simulink model "Realizacion_Retroalimentacion_Estados"  (R2023b)
settings: Solver=ode4  StartTime=0.0  StopTime=15  FixedStep=0.01  RelTol=1e-3
values from neighbouring files (symbols this model uses):
  Gf = feedback(G1*G2,H)    [Exp1_Realizacion.m]
  K = place(A,B,pcc)    [Exp1_Realizacion.m]
  Ke = Ke'    [Exp1_Realizacion.m]
undefined symbols (not defined in the file or in its folder): A, B, C, D
settings Model: Creator=carlo  LastModifiedBy=carlo

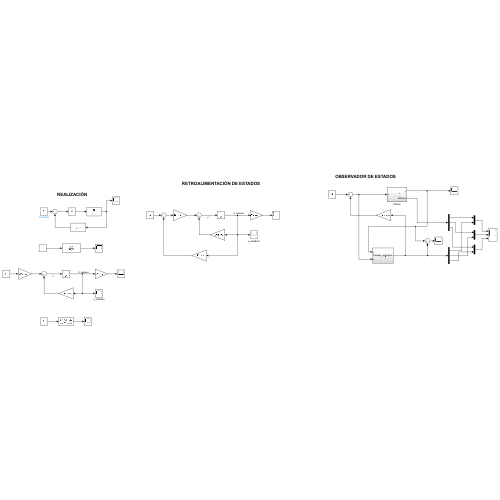
[thumbnail: Simulink's stored preview of the top-level diagram]
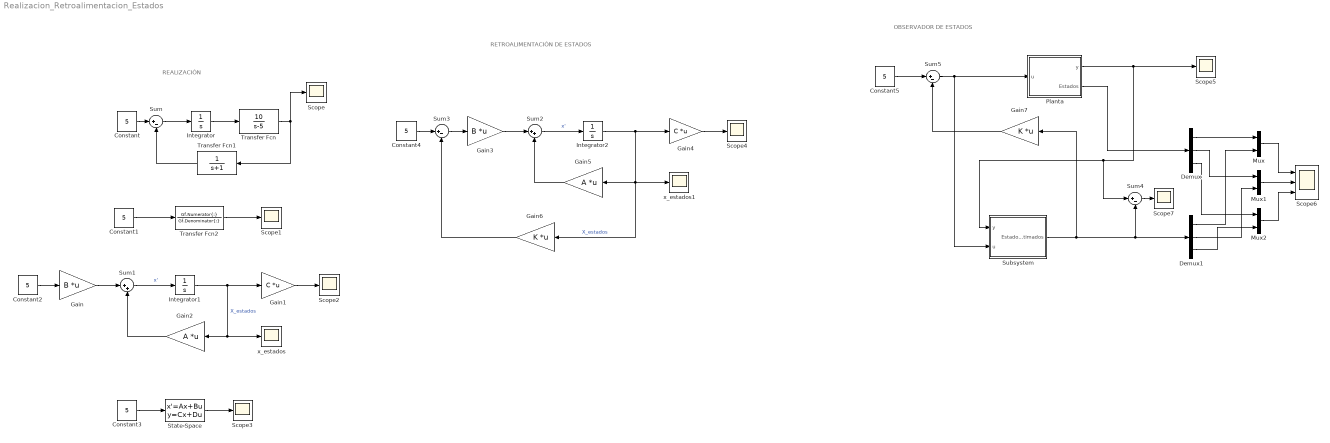
== system Realizacion_Retroalimentacion_Estados ==
  note: REALIZACIÓN
  note: RETROALIMENTACIÓN DE ESTADOS
  note: OBSERVADOR DE ESTADOS
  Constant{,1..5} (6 alike) : Constant  Value=5
  Demux : Demux  Outputs=3
  Demux1 : Demux  Outputs=3
  Gain : Gain  Gain=B  Multiplication=Matrix(K*u) (u vector)
  Gain1 : Gain  Gain=C  Multiplication=Matrix(K*u) (u vector)
  Gain2 : Gain  Gain=A  Multiplication=Matrix(K*u) (u vector)
  Gain3 : Gain  Gain=B  Multiplication=Matrix(K*u) (u vector)
  Gain4 : Gain  Gain=C  Multiplication=Matrix(K*u) (u vector)
  Gain5 : Gain  Gain=A  Multiplication=Matrix(K*u) (u vector)
  Gain6 : Gain  Gain=K  Multiplication=Matrix(K*u) (u vector)
  Gain7 : Gain  Gain=K  Multiplication=Matrix(K*u) (u vector)
  Integrator : Integrator
  Integrator1 : Integrator  InitialCondition=[2 4 7]'
  Integrator2 : Integrator  InitialCondition=[5 -4 7]'
  Mux : Mux  Inputs=2
  Mux1 : Mux  Inputs=2
  Mux2 : Mux  Inputs=2
  Planta : Subsystem
  Scope{,1..5,7} (7 alike) : Scope
  Scope6 : Scope  NumInputPorts=3
  State-Space : StateSpace  A=A  B=B  C=C  D=D  InitialCondition=[3 0 0]'
  Subsystem : Subsystem
  Sum{,3..5} (4 alike) : Sum  Inputs=|+-
  Sum1 : Sum  Inputs=|++
  Sum2 : Sum  Inputs=|++
  Transfer Fcn : TransferFcn  Numerator=[10]  Denominator=[1 -5]
  Transfer Fcn1 : TransferFcn  Denominator=[1 1]
  Transfer Fcn2 : TransferFcn  Numerator=Gf.Numerator{:}  Denominator=Gf.Denominator{:}
  x_estados : Scope
  x_estados1 : Scope
  wires:
  Constant/1 -> Sum/1
  Sum/1 -> Integrator/1
  Integrator/1 -> Transfer Fcn/1
  Transfer Fcn/1 -> Scope/1, Transfer Fcn1/1
  Transfer Fcn1/1 -> Sum/2
  Constant1/1 -> Transfer Fcn2/1
  Transfer Fcn2/1 -> Scope1/1
  Gain2/1 -> Sum1/2
  Integrator1/1 -> x_estados/1, Gain2/1, Gain1/1  "X_estados"
  Gain/1 -> Sum1/1
  Sum1/1 -> Integrator1/1  "x'"
  Constant2/1 -> Gain/1
  Gain1/1 -> Scope2/1
  Constant3/1 -> State-Space/1
  State-Space/1 -> Scope3/1
  Gain4/1 -> Scope4/1
  Sum2/1 -> Integrator2/1  "x'"
  Gain3/1 -> Sum2/1
  Integrator2/1 -> Gain4/1, Gain6/1, x_estados1/1, Gain5/1  "X_estados"
  Gain5/1 -> Sum2/2
  Constant4/1 -> Sum3/1
  Sum3/1 -> Gain3/1
  Gain6/1 -> Sum3/2
  Constant5/1 -> Sum5/1
  Sum5/1 -> Subsystem/2(u), Planta/1(u)
  Planta/1(y) -> Sum4/1, Subsystem/1(y), Scope5/1
  Subsystem/1(Estados_estimados) -> Gain7/1, Sum4/2, Demux1/1
  Planta/2(Estados) -> Demux/1
  Demux/1 -> Mux/1
  Demux1/1 -> Mux/2
  Demux/2 -> Mux1/1
  Demux1/2 -> Mux1/2
  Demux/3 -> Mux2/1
  Demux1/3 -> Mux2/2
  Mux/1 -> Scope6/1
  Mux1/1 -> Scope6/2
  Mux2/1 -> Scope6/3
  Gain7/1 -> Sum5/2
  Sum4/1 -> Scope7/1

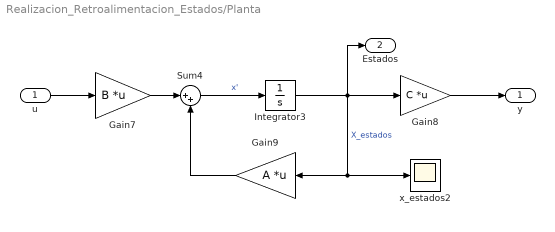
== system Realizacion_Retroalimentacion_Estados/Planta ==
  u : Inport
  Gain7 : Gain  Gain=B  Multiplication=Matrix(K*u) (u vector)
  Gain8 : Gain  Gain=C  Multiplication=Matrix(K*u) (u vector)
  Gain9 : Gain  Gain=A  Multiplication=Matrix(K*u) (u vector)
  Integrator3 : Integrator  InitialCondition=[-10 0 35]'
  Sum4 : Sum  Inputs=|++
  x_estados2 : Scope
  y : Outport
  Estados : Outport  Port=2
  wires:
  Sum4/1 -> Integrator3/1  "x'"
  Gain7/1 -> Sum4/1
  Integrator3/1 -> Estados/1, x_estados2/1, Gain9/1, Gain8/1  "X_estados"
  Gain8/1 -> y/1
  Gain9/1 -> Sum4/2
  u/1 -> Gain7/1

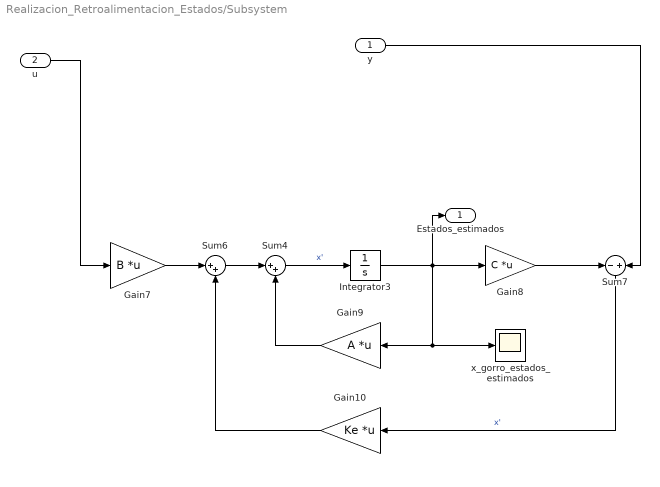
== system Realizacion_Retroalimentacion_Estados/Subsystem ==
  y : Inport
  u : Inport  Port=2
  Gain10 : Gain  Gain=Ke  Multiplication=Matrix(K*u) (u vector)
  Gain7 : Gain  Gain=B  Multiplication=Matrix(K*u) (u vector)
  Gain8 : Gain  Gain=C  Multiplication=Matrix(K*u) (u vector)
  Gain9 : Gain  Gain=A  Multiplication=Matrix(K*u) (u vector)
  Integrator3 : Integrator  InitialCondition=[0 0 0]'
  Sum4 : Sum  Inputs=|++
  Sum6 : Sum  Inputs=|++
  Sum7 : Sum  Inputs=-+
  x_gorro_estados_estimados : Scope
  Estados_estimados : Outport
  wires:
  Sum4/1 -> Integrator3/1  "x'"
  Sum6/1 -> Sum4/1
  Integrator3/1 -> Estados_estimados/1, x_gorro_estados_estimados/1, Gain9/1, Gain8/1
  Gain10/1 -> Sum6/2
  Sum7/1 -> Gain10/1  "x'"
  Gain9/1 -> Sum4/2
  Gain8/1 -> Sum7/1
  Gain7/1 -> Sum6/1
  u/1 -> Gain7/1
  y/1 -> Sum7/2
